simulink model "SIM_SAD_DEMO"  (R2025b)
settings: Solver=ode5  StartTime=0.0  StopTime=2*T  FixedStep=0.1  RelTol=1e-3
model workspace (MAT data in the model file):
  Pnull : Simulink.Parameter (value not decoded)
  rho_albedo_medio : Simulink.Parameter (value not decoded)
values from neighbouring files (symbols this model uses):
  Aree = zeros(10,1)    [SCRIPT_SAD_DEMO.m]
  base_seed = base_seed_MC + k    [SCRIPT_SAD_DEMO.m]
  c = astroConstants(5)*1e3    [SCRIPT_SAD_DEMO.m]
  draan = 1.99096871e-7    (= 1.99096871e-07)    [SCRIPT_SAD_DEMO.m]
  dwell_time = 30    [SCRIPT_SAD_DEMO.m]
  eps_att = deg2rad(0.2)    [SCRIPT_SAD_DEMO.m]
  eps_E = deg2rad(astroConstants(63))    [SCRIPT_SAD_DEMO.m]
  eps_h_r = 0.001    [SCRIPT_SAD_DEMO.m]
  eps_w = deg2rad(0.1)    [SCRIPT_SAD_DEMO.m]
  err_max = deg2rad(15)    [SCRIPT_SAD_DEMO.m]
  F_e = 1358    [SCRIPT_SAD_DEMO.m]
  h_r_max = 0.05    [SCRIPT_SAD_DEMO.m]
  h_r_safe = 0.001    [SCRIPT_SAD_DEMO.m]
  j_B = [0.01; 0.05; 0.01]    [SCRIPT_SAD_DEMO.m]
  J_depl = J_nom    [SCRIPT_SAD_DEMO.m]
  JD0 = juliandate(startTime)    [SCRIPT_SAD_DEMO.m]
  k_b = 200000    [SCRIPT_SAD_DEMO.m]
  Kd = K(:, 1:3)    [SCRIPT_SAD_DEMO.m]
  kep = [a,e,incl,raan,w,theta]    [SCRIPT_SAD_DEMO.m]
  Kp = K(:, 4:6)    [SCRIPT_SAD_DEMO.m]
  mu = astroConstants(13)    [SCRIPT_SAD_DEMO.m]
  n = sqrt( (mu/ (a)^3))    [SCRIPT_SAD_DEMO.m]
  n_sun = 2*pi/T_sun    (= 1.99238499086e-07)    [SCRIPT_SAD_DEMO.m]
  Nmat = [ ... (first row only)    [SCRIPT_SAD_DEMO.m]
  r_sun = 1*AU    [SCRIPT_SAD_DEMO.m]
  Re = astroConstants(23)    [SCRIPT_SAD_DEMO.m]
  rf = [ ... (first row only)    [SCRIPT_SAD_DEMO.m]
  rhod = 0.1*ones(10,1)    [SCRIPT_SAD_DEMO.m]
  rhos = zeros(10,1)    [SCRIPT_SAD_DEMO.m]
  SRP = SRP_nom    [SCRIPT_SAD_DEMO.m]
  theta = 0    [SCRIPT_SAD_DEMO.m]
  w0 = w0_nom    [SCRIPT_SAD_DEMO.m]
  w_enter = Control.w_tumbling    [SCRIPT_SAD_DEMO.m]
  w_enter_2 = Control.w_pointing    [SCRIPT_SAD_DEMO.m]
  w_exit = deg2rad(4)    [SCRIPT_SAD_DEMO.m]
  w_exit_2 = deg2rad(1.5)    [SCRIPT_SAD_DEMO.m]
symbols that are objects in the model workspace (value not decoded): Pnull, rho_albedo_medio
undefined symbols (not defined in the file or in its folder): DiscIntNeverNeededParam, Filter, Gyro, Magmeter, MTQ, q, RW, Sun_sensor
libraries: matrix_library x41, LIBRARY_SAD x40, simulink x1, cstblocks x1
(part 3 of 4)

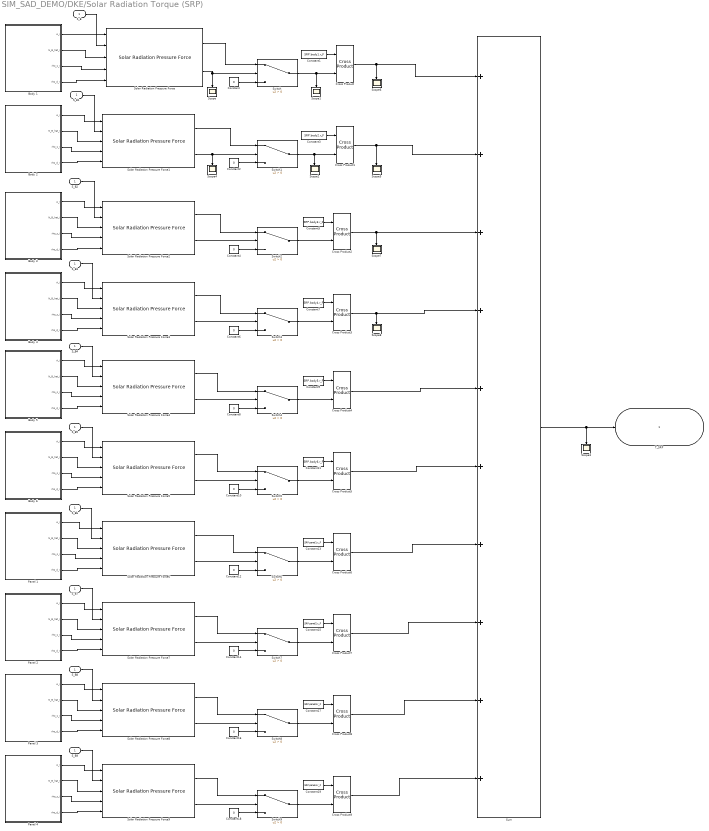
== system SIM_SAD_DEMO/DKE/Solar Radiation Torque (SRP) ==
  S_B : Inport
  Body 1 : Subsystem
  Body 2 : Subsystem
  Body 3 : Subsystem
  Body 4 : Subsystem
  Body 5 : Subsystem
  Body 6 : Subsystem
  Constant{,2,4,6,8,10,12,14,16,18} (10 alike) : Constant  Value=0
  Constant1 : Constant  Value=SRP.body1.r_F
  Constant11 : Constant  Value=SRP.body6.r_F
  Constant13 : Constant  Value=SRP.panel1.r_F
  Constant15 : Constant  Value=SRP.panel2.r_F
  Constant17 : Constant  Value=SRP.panel3.r_F
  Constant19 : Constant  Value=SRP.panel4.r_F
  Constant3 : Constant  Value=SRP.body2.r_F
  Constant5 : Constant  Value=SRP.body3.r_F
  Constant7 : Constant  Value=SRP.body4.r_F
  Constant9 : Constant  Value=SRP.body5.r_F
  Cross Product{,1..9} (10 alike) : matrix_library/Cross Product
  Panel 1 : Subsystem
  Panel 2 : Subsystem
  Panel 3 : Subsystem
  Panel 4 : Subsystem
  S_B{1..9} (9 alike) : InportShadow
  Scope{,1..8} (9 alike) : Scope
      Scope settings: ActiveDisplayYMinimum=-1  ActiveDisplayYMaximum=1  DataLoggingVariableName=ScopeData9
      Scope1 settings: ActiveDisplayYMinimum=-1  ActiveDisplayYMaximum=1  DataLoggingVariableName=ScopeData10
      Scope2 settings: ActiveDisplayYMinimum=-1  ActiveDisplayYMaximum=1  DataLoggingVariableName=ScopeData11
      Scope3 settings: ActiveDisplayYMinimum=-5.1359030627651383E-25  ActiveDisplayYMaximum=9.2718061255302776E-25  DataLoggingVariableName=ScopeData12
      Scope4 settings: ActiveDisplayYMinimum=-1  ActiveDisplayYMaximum=1  DataLoggingVariableName=ScopeData13
      Scope5 settings: ActiveDisplayYMinimum=-1  ActiveDisplayYMaximum=1  DataLoggingVariableName=ScopeData14
      Scope6 settings: ActiveDisplayYMinimum=-1  ActiveDisplayYMaximum=1  DataLoggingVariableName=ScopeData15
      Scope7 settings: ActiveDisplayYMinimum=-1  ActiveDisplayYMaximum=1  DataLoggingVariableName=ScopeData18
      Scope8 settings: ActiveDisplayYMinimum=-1  ActiveDisplayYMaximum=1  DataLoggingVariableName=ScopeData19
  Solar Radiation Pressure Force{,1..9} (10 alike) : LIBRARY_SAD/Solar Radiation Pressure Force  SystemSampleTime=-1  VariantActivationTime=update diagram  EmptyChoice=off  PassThrough=off  PassThroughVariantControl=(default)  EmptyChoiceVariantControl=(default)  AllowFlexibleInterface=on  Latency=0  AutoFrameSizeCalculation=off
  Sum : Sum  Inputs=++++++++++
  Switch{,1..9} (10 alike) : Switch  Criteria=u2 > Threshold  SaturateOnIntegerOverflow=off  InputSameDT=off
  T_SRP : Outport
  wires:
  S_B/1 -> Solar Radiation Pressure Force/2
  Body 1/1(A_i) -> Solar Radiation Pressure Force/1
  Body 1/2(N_B_hat_i) -> Solar Radiation Pressure Force/3
  Body 1/3(rho_s_i) -> Solar Radiation Pressure Force/4
  Body 1/4(rho_d_i) -> Solar Radiation Pressure Force/5
  Solar Radiation Pressure Force/1 -> Switch/1
  Solar Radiation Pressure Force/2 -> Scope/1, Switch/2
  Body 2/4(rho_d_i) -> Solar Radiation Pressure Force1/5
  Body 2/3(rho_s_i) -> Solar Radiation Pressure Force1/4
  Body 2/2(N_B_hat_i) -> Solar Radiation Pressure Force1/3
  Body 2/1(A_i) -> Solar Radiation Pressure Force1/1
  S_B1/1 -> Solar Radiation Pressure Force1/2
  S_B2/1 -> Solar Radiation Pressure Force2/2
  Body 3/1(A_i) -> Solar Radiation Pressure Force2/1
  Body 3/2(N_B_hat_i) -> Solar Radiation Pressure Force2/3
  Body 3/3(rho_s_i) -> Solar Radiation Pressure Force2/4
  Body 3/4(rho_d_i) -> Solar Radiation Pressure Force2/5
  Body 4/4(rho_d_i) -> Solar Radiation Pressure Force3/5
  Body 4/3(rho_s_i) -> Solar Radiation Pressure Force3/4
  Body 4/2(N_B_hat_i) -> Solar Radiation Pressure Force3/3
  Body 4/1(A_i) -> Solar Radiation Pressure Force3/1
  S_B3/1 -> Solar Radiation Pressure Force3/2
  S_B4/1 -> Solar Radiation Pressure Force4/2
  Body 5/1(A_i) -> Solar Radiation Pressure Force4/1
  Body 5/2(N_B_hat_i) -> Solar Radiation Pressure Force4/3
  Body 5/3(rho_s_i) -> Solar Radiation Pressure Force4/4
  Body 5/4(rho_d_i) -> Solar Radiation Pressure Force4/5
  Body 6/4(rho_d_i) -> Solar Radiation Pressure Force5/5
  Body 6/3(rho_s_i) -> Solar Radiation Pressure Force5/4
  Body 6/2(N_B_hat_i) -> Solar Radiation Pressure Force5/3
  Body 6/1(A_i) -> Solar Radiation Pressure Force5/1
  S_B5/1 -> Solar Radiation Pressure Force5/2
  S_B6/1 -> Solar Radiation Pressure Force6/2
  Panel 1/1(A_i) -> Solar Radiation Pressure Force6/1
  Panel 1/2(N_B_hat_i) -> Solar Radiation Pressure Force6/3
  Panel 1/3(rho_s_i) -> Solar Radiation Pressure Force6/4
  Panel 1/4(rho_d_i) -> Solar Radiation Pressure Force6/5
  Panel 2/4(rho_d_i) -> Solar Radiation Pressure Force7/5
  Panel 2/3(rho_s_i) -> Solar Radiation Pressure Force7/4
  Panel 2/2(N_B_hat_i) -> Solar Radiation Pressure Force7/3
  Panel 2/1(A_i) -> Solar Radiation Pressure Force7/1
  S_B7/1 -> Solar Radiation Pressure Force7/2
  S_B8/1 -> Solar Radiation Pressure Force8/2
  Panel 3/1(A_i) -> Solar Radiation Pressure Force8/1
  Panel 3/2(N_B_hat_i) -> Solar Radiation Pressure Force8/3
  Panel 3/3(rho_s_i) -> Solar Radiation Pressure Force8/4
  Panel 3/4(rho_d_i) -> Solar Radiation Pressure Force8/5
  Panel 4/4(rho_d_i) -> Solar Radiation Pressure Force9/5
  Panel 4/3(rho_s_i) -> Solar Radiation Pressure Force9/4
  Panel 4/2(N_B_hat_i) -> Solar Radiation Pressure Force9/3
  Panel 4/1(A_i) -> Solar Radiation Pressure Force9/1
  S_B9/1 -> Solar Radiation Pressure Force9/2
  Constant/1 -> Switch/3
  Switch/1 -> Scope1/1, Cross Product/2
  Constant1/1 -> Cross Product/1
  Cross Product/1 -> Scope6/1, Sum/1
  Cross Product1/1 -> Sum/2, Scope5/1
  Constant3/1 -> Cross Product1/1
  Switch1/1 -> Scope2/1, Cross Product1/2
  Constant2/1 -> Switch1/3
  Solar Radiation Pressure Force1/2 -> Scope4/1, Switch1/2
  Solar Radiation Pressure Force1/1 -> Switch1/1
  Solar Radiation Pressure Force2/1 -> Switch2/1
  Solar Radiation Pressure Force2/2 -> Switch2/2
  Constant4/1 -> Switch2/3
  Switch2/1 -> Cross Product2/2
  Constant5/1 -> Cross Product2/1
  Cross Product2/1 -> Scope7/1, Sum/3
  Cross Product3/1 -> Scope8/1, Sum/4
  Constant7/1 -> Cross Product3/1
  Switch3/1 -> Cross Product3/2
  Constant6/1 -> Switch3/3
  Solar Radiation Pressure Force3/2 -> Switch3/2
  Solar Radiation Pressure Force3/1 -> Switch3/1
  Solar Radiation Pressure Force4/1 -> Switch4/1
  Solar Radiation Pressure Force4/2 -> Switch4/2
  Constant8/1 -> Switch4/3
  Switch4/1 -> Cross Product4/2
  Constant9/1 -> Cross Product4/1
  Cross Product4/1 -> Sum/5
  Cross Product5/1 -> Sum/6
  Constant11/1 -> Cross Product5/1
  Switch5/1 -> Cross Product5/2
  Constant10/1 -> Switch5/3
  Solar Radiation Pressure Force5/2 -> Switch5/2
  Solar Radiation Pressure Force5/1 -> Switch5/1
  Solar Radiation Pressure Force6/1 -> Switch6/1
  Solar Radiation Pressure Force6/2 -> Switch6/2
  Constant12/1 -> Switch6/3
  Switch6/1 -> Cross Product6/2
  Constant13/1 -> Cross Product6/1
  Cross Product6/1 -> Sum/7
  Cross Product7/1 -> Sum/8
  Constant15/1 -> Cross Product7/1
  Switch7/1 -> Cross Product7/2
  Constant14/1 -> Switch7/3
  Solar Radiation Pressure Force7/2 -> Switch7/2
  Solar Radiation Pressure Force7/1 -> Switch7/1
  Solar Radiation Pressure Force8/1 -> Switch8/1
  Solar Radiation Pressure Force8/2 -> Switch8/2
  Constant16/1 -> Switch8/3
  Switch8/1 -> Cross Product8/2
  Constant17/1 -> Cross Product8/1
  Cross Product8/1 -> Sum/9
  Cross Product9/1 -> Sum/10
  Constant19/1 -> Cross Product9/1
  Switch9/1 -> Cross Product9/2
  Constant18/1 -> Switch9/3
  Solar Radiation Pressure Force9/2 -> Switch9/2
  Solar Radiation Pressure Force9/1 -> Switch9/1
  Sum/1 -> Scope3/1, T_SRP/1

== system SIM_SAD_DEMO/DKE/Sun-Earth Orbit ==
  Clock : Clock
  Clock1 : Clock
  Clock2 : Clock
  Constant : Constant  Value=n_sun
  Constant1 : Constant  Value=eps_E
  Constant2 : Constant  Value=r_sun
  Constant3 : Constant  Value=n_sun
  Constant4 : Constant  Value=eps_E
  Constant5 : Constant  Value=n_sun
  Cos : Trigonometry  Operator=cos
  Cos1 : Trigonometry  Operator=cos
  Cos2 : Trigonometry
  Product{,1..5} (6 alike) : Product
  Sin : Trigonometry
  Sin1 : Trigonometry
  Vector Concatenate : Concatenate  NumInputs=3
  r_Sun_N : Outport
  wires:
  Constant2/1 -> Product/1
  Clock/1 -> Product1/1
  Constant/1 -> Product1/2
  Product1/1 -> Cos/1
  Cos/1 -> Vector Concatenate/1
  Product2/1 -> Sin/1
  Constant3/1 -> Product2/2
  Clock1/1 -> Product2/1
  Sin/1 -> Product3/1
  Constant1/1 -> Cos1/1
  Product3/1 -> Vector Concatenate/2
  Cos1/1 -> Product3/2
  Cos2/1 -> Product5/2
  Product5/1 -> Vector Concatenate/3
  Constant4/1 -> Cos2/1
  Sin1/1 -> Product5/1
  Clock2/1 -> Product4/1
  Constant5/1 -> Product4/2
  Product4/1 -> Sin1/1
  Vector Concatenate/1 -> Product/2
  Product/1 -> r_Sun_N/1

== system SIM_SAD_DEMO/DKE/w_LVLH//N ==
  theta_dot : Inport
  Constant2 : Constant  Value=0
  Constant3 : Constant  Value=0
  Vector Concatenate1 : Concatenate  NumInputs=3
  Out1 : Outport
  wires:
  Vector Concatenate1/1 -> Out1/1  "w_LVLH/N"
  Constant2/1 -> Vector Concatenate1/1
  Constant3/1 -> Vector Concatenate1/2
  theta_dot/1 -> Vector Concatenate1/3

== system SIM_SAD_DEMO/SENSORS/Gyroscope ==
  note: Misalignment e non-orthogonality
  note: Scale Factor Errors
  w_B (rad/s) : Inport
  Abs : Abs  SaturateOnIntegerOverflow=off
  Bias Instability (Brown noise) : RandomNumber  Seed=base_seed + 10  SampleTime=0.2
  Constant : Constant  Value=Gyro.R
  Constant1 : Constant  Value=Gyro.O
  Constant2 : Constant  Value=Gyro.b
  Constant3 : Constant  Value=0
  D2R : Gain  Gain=pi/180
  Discrete-Time Integrator : DiscreteIntegrator  SampleTime=-1  ICPrevOutput=DiscIntNeverNeededParam  ICPrevScaledInput=DiscIntNeverNeededParam
  Gain2 : Gain  Gain=Gyro.D/(sqrt(2*Gyro.Ts))
  Gain4 : Gain  Gain=Gyro.D/(sqrt(2*Gyro.Ts))
  Gain5 : Gain  Gain=1/Gyro.ctime
  Gain6 : Gain  Gain=Gyro.NL/100
  MatrixMultiply : Product  Multiplication=Matrix(*)
  MatrixMultiply2 : Product  Multiplication=Matrix(*)
  Minus : Sum  Inputs=+-
  Plus : Sum
  Plus1 : Sum  Inputs=+++
  Plus2 : Sum
  Quantizer : Quantizer  QuantizationInterval=Gyro.LSB
  R2D : Gain  Gain=180/pi
  R2D_1 : Gain  Gain=180/pi
  Saturation : Saturate  UpperLimit=Gyro.FS/2  LowerLimit=-Gyro.FS/2
  Scope{,1..6} (7 alike) : Scope
      Scope settings: ActiveDisplayYMinimum=-1  ActiveDisplayYMaximum=1  DataLoggingVariableName=ScopeData38
      Scope1 settings: ActiveDisplayYMinimum=-1  ActiveDisplayYMaximum=1  DataLoggingVariableName=ScopeData39
      Scope2 settings: ActiveDisplayYMinimum=-1  ActiveDisplayYMaximum=1  DataLoggingVariableName=ScopeData40
      Scope3 settings: ActiveDisplayYMinimum=-1  ActiveDisplayYMaximum=1  DataLoggingVariableName=ScopeData41
      Scope4 settings: ActiveDisplayYMinimum=-1  ActiveDisplayYMaximum=1  DataLoggingVariableName=ScopeData42
      Scope5 settings: ActiveDisplayYMinimum=-0.14265311547660356  ActiveDisplayYMaximum=1.1268108470363587  DataLoggingVariableName=ScopeData43
      Scope6 settings: ActiveDisplayYMinimum=-0.12498036504591503  ActiveDisplayYMaximum=1.124997818338435  DataLoggingVariableName=ScopeData44
  Square : Math  Operator=square
  Switch : Switch  Criteria=u2 > Threshold  Threshold=2*Gyro.NL*Gyro.FS  SaturateOnIntegerOverflow=off  InputSameDT=off
  White noise : RandomNumber  Seed=base_seed + 9  SampleTime=0.2
  Zero-Order Hold : ZeroOrderHold  SampleTime=Gyro.Ts
  w_m : Outport
  wires:
  w_B (rad/s)/1 -> MatrixMultiply/2, R2D_1/1
  MatrixMultiply/1 -> MatrixMultiply2/2
  Constant/1 -> MatrixMultiply/1, Scope5/1
  Constant1/1 -> Scope6/1, MatrixMultiply2/1
  MatrixMultiply2/1 -> R2D/1
  Constant2/1 -> Plus1/1
  Plus1/1 -> Scope4/1, Quantizer/1
  Quantizer/1 -> Saturation/1
  Saturation/1 -> D2R/1
  Zero-Order Hold/1 -> w_m/1
  D2R/1 -> Zero-Order Hold/1
  White noise/1 -> Gain2/1
  Bias Instability (Brown noise)/1 -> Gain4/1
  Gain2/1 -> Plus2/1, Scope2/1
  Gain4/1 -> Minus/1
  Minus/1 -> Discrete-Time Integrator/1
  Abs/1 -> Switch/2
  Square/1 -> Gain6/1
  Gain6/1 -> Switch/1
  Constant3/1 -> Switch/3
  R2D_1/1 -> Abs/1, Square/1
  Switch/1 -> Scope1/1, Plus/2
  Gain5/1 -> Minus/2
  Plus2/1 -> Scope3/1, Plus1/3
  Discrete-Time Integrator/1 -> Plus2/2, Gain5/1
  Plus/1 -> Plus1/2
  R2D/1 -> Plus/1, Scope/1

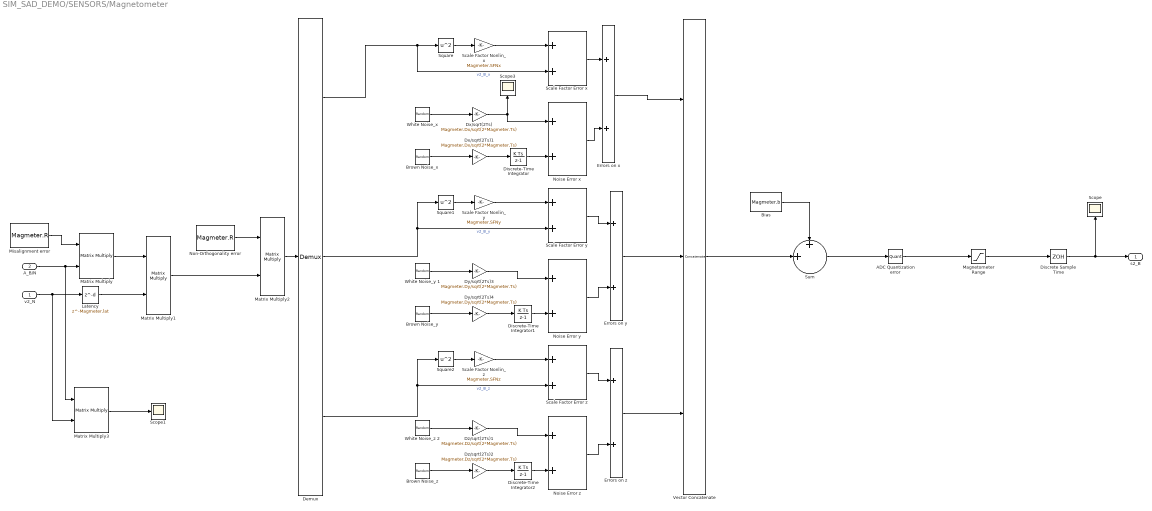
== system SIM_SAD_DEMO/SENSORS/Magnetometer ==
  v2_N : Inport
  A_B/N : Inport  Port=2
  ADC Quantization error : Quantizer  QuantizationInterval=Magmeter.LSB
  Bias : Constant  Value=Magmeter.b
  Brown Noise_x : RandomNumber  Seed=base_seed + 4  SampleTime=0.1
  Brown Noise_y : RandomNumber  Seed=base_seed + 6  SampleTime=0.1
  Brown Noise_z : RandomNumber  Seed=base_seed + 8  SampleTime=0.1
  Demux : Demux  Outputs=3
  Discrete Sample Time : ZeroOrderHold  SampleTime=Magmeter.Ts
  Discrete-Time Integrator : DiscreteIntegrator  SampleTime=-1  ICPrevOutput=DiscIntNeverNeededParam  ICPrevScaledInput=DiscIntNeverNeededParam
  Discrete-Time Integrator1 : DiscreteIntegrator  SampleTime=-1  ICPrevOutput=DiscIntNeverNeededParam  ICPrevScaledInput=DiscIntNeverNeededParam
  Discrete-Time Integrator2 : DiscreteIntegrator  SampleTime=-1  ICPrevOutput=DiscIntNeverNeededParam  ICPrevScaledInput=DiscIntNeverNeededParam
  Dx/sqrt(2Ts) : Gain  Gain=Magmeter.Dx/sqrt(2*Magmeter.Ts)
  Dx/sqrt(2Ts)1 : Gain  Gain=Magmeter.Dx/sqrt(2*Magmeter.Ts)
  Dy/sqrt(2Ts)3 : Gain  Gain=Magmeter.Dy/sqrt(2*Magmeter.Ts)
  Dy/sqrt(2Ts)4 : Gain  Gain=Magmeter.Dy/sqrt(2*Magmeter.Ts)
  Dz/sqrt(2Ts)1 : Gain  Gain=Magmeter.Dz/sqrt(2*Magmeter.Ts)
  Dz/sqrt(2Ts)2 : Gain  Gain=Magmeter.Dz/sqrt(2*Magmeter.Ts)
  Errors on x : Sum
  Errors on y : Sum
  Errors on z : Sum
  Latency : Delay  DelayLength=Magmeter.lat
  Magnetometer Range : Saturate  UpperLimit=Magmeter.FS(2)  LowerLimit=Magmeter.FS(1)
  Matrix Multiply{,1..3} (4 alike) : Product  Multiplication=Matrix(*)
  Misalignment error : Constant  Value=Magmeter.R
  Noise Error x : Sum
  Noise Error y : Sum
  Noise Error z : Sum
  Non-Orthogonality error : Constant  Value=Magmeter.R
  Scale Factor Error x : Sum
  Scale Factor Error y : Sum
  Scale Factor Error z : Sum
  Scale Factor Nonlin_x : Gain  Gain=Magmeter.SFNx
  Scale Factor Nonlin_y : Gain  Gain=Magmeter.SFNy
  Scale Factor Nonlin_z : Gain  Gain=Magmeter.SFNz
  Scope : Scope
      settings: ActiveDisplayYMinimum=-2.19268798828125E-5  ActiveDisplayYMaximum=3.19366455078125E-5  DataLoggingVariableName=ScopeData41
  Scope1 : Scope
      settings: ActiveDisplayYMinimum=-2.3197965857438213E-5  ActiveDisplayYMaximum=2.9408763146413098E-5  DataLoggingVariableName=ScopeData51
  Scope3 : Scope
      settings: ActiveDisplayYMinimum=-2.2049299467588538E-7  ActiveDisplayYMaximum=2.2303254095659386E-7  DataLoggingVariableName=ScopeData59
  Square : Math  Operator=square
  Square1 : Math  Operator=square
  Square2 : Math  Operator=square
  Sum : Sum  Inputs=++|
  Vector Concatenate : Concatenate  NumInputs=3
  "White Noise_x " : RandomNumber  Seed=base_seed + 3  SampleTime=0.1
  White Noise_y 1 : RandomNumber  Seed=base_seed + 5  SampleTime=0.1
  White Noise_z 2 : RandomNumber  Seed=base_seed + 7  SampleTime=0.1
  s2_B : Outport
  wires:
  v2_N/1 -> Matrix Multiply3/2, Latency/1
  A_B/N/1 -> Matrix Multiply3/1, Matrix Multiply/2
  Matrix Multiply/1 -> Matrix Multiply1/1
  Misalignment error/1 -> Matrix Multiply/1
  Latency/1 -> Matrix Multiply1/2
  Matrix Multiply1/1 -> Matrix Multiply2/2
  Non-Orthogonality error/1 -> Matrix Multiply2/1
  Matrix Multiply2/1 -> Demux/1
  Demux/1 -> Square/1, Scale Factor Error x/2  "v2_B_x"
  Demux/2 -> Square1/1, Scale Factor Error y/2  "v2_B_y"
  "White Noise_x "/1 -> Dx/sqrt(2Ts)/1
  Square/1 -> Scale Factor Nonlin_x/1
  Scale Factor Nonlin_x/1 -> Scale Factor Error x/1
  Noise Error x/1 -> Errors on x/2
  Scale Factor Error x/1 -> Errors on x/1
  Bias/1 -> Sum/1
  Errors on x/1 -> Vector Concatenate/1
  Vector Concatenate/1 -> Sum/2
  Sum/1 -> ADC Quantization error/1
  ADC Quantization error/1 -> Magnetometer Range/1
  Magnetometer Range/1 -> Discrete Sample Time/1
  Discrete Sample Time/1 -> s2_B/1, Scope/1
  Brown Noise_x/1 -> Dx/sqrt(2Ts)1/1
  Discrete-Time Integrator/1 -> Noise Error x/2
  Dx/sqrt(2Ts)1/1 -> Discrete-Time Integrator/1
  Demux/3 -> Scale Factor Error z/2, Square2/1  "v2_B_z"
  Dy/sqrt(2Ts)4/1 -> Discrete-Time Integrator1/1
  Discrete-Time Integrator1/1 -> Noise Error y/2
  Brown Noise_y/1 -> Dy/sqrt(2Ts)4/1
  Errors on y/1 -> Vector Concatenate/2
  Dy/sqrt(2Ts)3/1 -> Noise Error y/1
  Scale Factor Error y/1 -> Errors on y/1
  Noise Error y/1 -> Errors on y/2
  Scale Factor Nonlin_y/1 -> Scale Factor Error y/1
  Square1/1 -> Scale Factor Nonlin_y/1
  White Noise_y 1/1 -> Dy/sqrt(2Ts)3/1
  White Noise_z 2/1 -> Dz/sqrt(2Ts)1/1
  Square2/1 -> Scale Factor Nonlin_z/1
  Scale Factor Nonlin_z/1 -> Scale Factor Error z/1
  Noise Error z/1 -> Errors on z/2
  Scale Factor Error z/1 -> Errors on z/1
  Dz/sqrt(2Ts)1/1 -> Noise Error z/1
  Errors on z/1 -> Vector Concatenate/3
  Brown Noise_z/1 -> Dz/sqrt(2Ts)2/1
  Discrete-Time Integrator2/1 -> Noise Error z/2
  Dz/sqrt(2Ts)2/1 -> Discrete-Time Integrator2/1
  Matrix Multiply3/1 -> Scope1/1
  Dx/sqrt(2Ts)/1 -> Scope3/1, Noise Error x/1

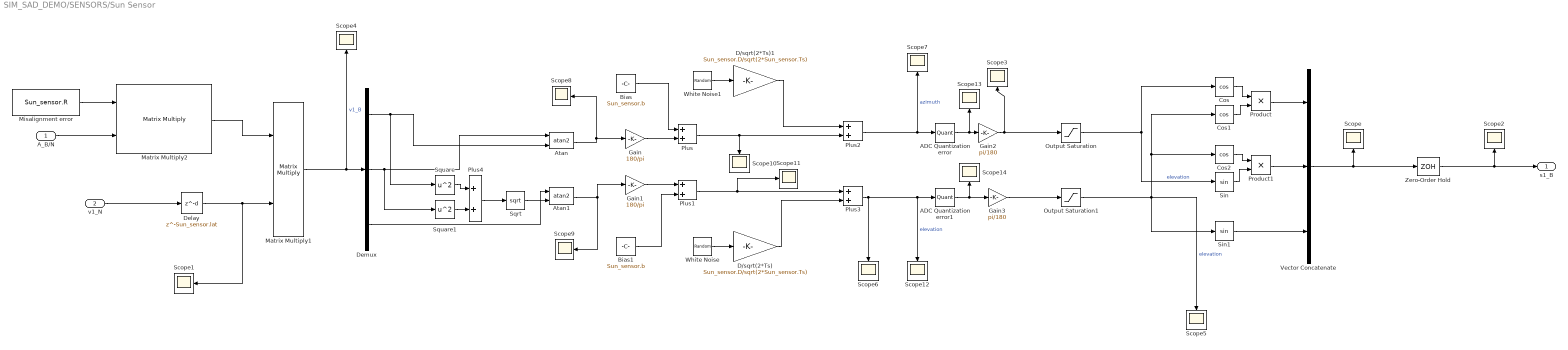
== system SIM_SAD_DEMO/SENSORS/Sun Sensor ==
  A_B/N : Inport
  v1_N : Inport  Port=2
  ADC Quantization error : Quantizer  QuantizationInterval=Sun_sensor.LSB
  ADC Quantization error1 : Quantizer  QuantizationInterval=Sun_sensor.LSB
  Atan : Trigonometry  Operator=atan2
  Atan1 : Trigonometry  Operator=atan2
  Bias : Constant  Value=Sun_sensor.b
  Bias1 : Constant  Value=Sun_sensor.b
  Cos : Trigonometry  Operator=cos
  Cos1 : Trigonometry  Operator=cos
  Cos2 : Trigonometry  Operator=cos
  D/sqrt(2*Ts) : Gain  Gain=Sun_sensor.D/sqrt(2*Sun_sensor.Ts)
  D/sqrt(2*Ts)1 : Gain  Gain=Sun_sensor.D/sqrt(2*Sun_sensor.Ts)
  Delay : Delay  DelayLength=Sun_sensor.lat
  Demux : Demux  Outputs=3
  Gain : Gain  Gain=180/pi
  Gain1 : Gain  Gain=180/pi
  Gain2 : Gain  Gain=pi/180
  Gain3 : Gain  Gain=pi/180
  Matrix Multiply1 : Product  Multiplication=Matrix(*)
  Matrix Multiply2 : Product  Multiplication=Matrix(*)
  Misalignment error : Constant  Value=Sun_sensor.R
  Output Saturation : Saturate  UpperLimit=Sun_sensor.FOV(2)  LowerLimit=Sun_sensor.FOV(1)
  Output Saturation1 : Saturate  UpperLimit=Sun_sensor.FOV(2)  LowerLimit=Sun_sensor.FOV(1)
  Plus{,1..4} (5 alike) : Sum
  Product : Product
  Product1 : Product
  Scope{,1..14} (15 alike) : Scope
      Scope settings: ActiveDisplayYMinimum=-1.2499999209761798  ActiveDisplayYMaximum=1.2499998658254696  DataLoggingVariableName=ScopeData38
      Scope1 settings: ActiveDisplayYMinimum=-0.50368682988878122  ActiveDisplayYMaximum=0.83961433978529221  DataLoggingVariableName=ScopeData39
      Scope10 settings: ActiveDisplayYMinimum=-1  ActiveDisplayYMaximum=1  DataLoggingVariableName=ScopeData48
      Scope11 settings: ActiveDisplayYMinimum=-0.16263647893928282  ActiveDisplayYMaximum=0.22803548611194213  DataLoggingVariableName=ScopeData49
      Scope12 settings: ActiveDisplayYMinimum=-1  ActiveDisplayYMaximum=1  DataLoggingVariableName=ScopeData50
      Scope13 settings: ActiveDisplayYMinimum=-225.30372619628906  ActiveDisplayYMaximum=225.44471740722656  DataLoggingVariableName=ScopeData53
      Scope14 settings: ActiveDisplayYMinimum=-0.908203125  ActiveDisplayYMaximum=0.95947265625  DataLoggingVariableName=ScopeData54
      Scope2 settings: ActiveDisplayYMinimum=-1.0615675808468883  ActiveDisplayYMaximum=1.1316838676859093  DataLoggingVariableName=ScopeData40
      Scope3 settings: ActiveDisplayYMinimum=-3.91845703125  ActiveDisplayYMaximum=3.91845703125  DataLoggingVariableName=ScopeData43
      Scope4 settings: ActiveDisplayYMinimum=-1.2500019852403355  ActiveDisplayYMaximum=1.2500020169480639  DataLoggingVariableName=ScopeData42
      Scope5 settings: ActiveDisplayYMinimum=-0.015851134808151625  ActiveDisplayYMaximum=0.01674595693441825  DataLoggingVariableName=ScopeData52
      Scope6 settings: ActiveDisplayYMinimum=-1  ActiveDisplayYMaximum=1  DataLoggingVariableName=ScopeData44
      Scope7 settings: ActiveDisplayYMinimum=-225.01352290442006  ActiveDisplayYMaximum=225.27088940788934  DataLoggingVariableName=ScopeData45
      Scope8 settings: ActiveDisplayYMinimum=-3.6715953390719882  ActiveDisplayYMaximum=3.318983817677017  DataLoggingVariableName=ScopeData46
      Scope9 settings: ActiveDisplayYMinimum=-1  ActiveDisplayYMaximum=1  DataLoggingVariableName=ScopeData47
  Sin : Trigonometry
  Sin1 : Trigonometry
  Sqrt : Sqrt
  Square : Math  Operator=square
  Square1 : Math  Operator=square
  Vector Concatenate : Concatenate  NumInputs=3
  White Noise : RandomNumber  Seed=base_seed + 2  SampleTime=0.1
  White Noise1 : RandomNumber  Seed=base_seed + 1  SampleTime=0.1
  Zero-Order Hold : ZeroOrderHold  SampleTime=Sun_sensor.Ts
  s1_B : Outport
  wires:
  A_B/N/1 -> Matrix Multiply2/2
  Zero-Order Hold/1 -> s1_B/1, Scope2/1
  Vector Concatenate/1 -> Zero-Order Hold/1, Scope/1
  v1_N/1 -> Delay/1
  Misalignment error/1 -> Matrix Multiply2/1
  White Noise/1 -> D/sqrt(2*Ts)/1
  Bias/1 -> Plus/1
  Matrix Multiply1/1 -> Scope4/1, Demux/1  "v1_B"
  Atan/1 -> Scope8/1, Gain/1
  Atan1/1 -> Gain1/1, Scope9/1
  Delay/1 -> Matrix Multiply1/2, Scope1/1
  Gain/1 -> Plus/2
  Gain1/1 -> Plus1/1
  Plus/1 -> Plus2/2, Scope10/1
  Plus1/1 -> Scope11/1, Plus3/1
  D/sqrt(2*Ts)/1 -> Plus3/2
  Bias1/1 -> Plus1/2
  White Noise1/1 -> D/sqrt(2*Ts)1/1
  D/sqrt(2*Ts)1/1 -> Plus2/1
  Demux/3 -> Atan1/1
  Demux/1 -> Square/1, Atan/2
  Product/1 -> Vector Concatenate/1
  Demux/2 -> Square1/1, Atan/1
  Square1/1 -> Plus4/2
  Square/1 -> Plus4/1
  Plus4/1 -> Sqrt/1
  Sqrt/1 -> Atan1/2
  Cos/1 -> Product/1
  Cos1/1 -> Product/2
  ADC Quantization error/1 -> Gain2/1, Scope13/1
  ADC Quantization error1/1 -> Gain3/1, Scope14/1
  Sin1/1 -> Vector Concatenate/3
  Cos2/1 -> Product1/1
  Sin/1 -> Product1/2
  Product1/1 -> Vector Concatenate/2
  Plus3/1 -> Scope6/1, ADC Quantization error1/1, Scope12/1  "elevation"
  Plus2/1 -> ADC Quantization error/1, Scope7/1  "azimuth"
  Matrix Multiply2/1 -> Matrix Multiply1/1
  Gain2/1 -> Scope3/1, Output Saturation/1
  Gain3/1 -> Output Saturation1/1
  Output Saturation/1 -> Cos/1, Sin/1  "elevation"
  Output Saturation1/1 -> Scope5/1, Cos2/1, Cos1/1, Sin1/1  "elevation"

== system SIM_SAD_DEMO/q-->DCM/[qΛ] ==
  q : Inport
  Constant : Constant  Value=0
  Constant1 : Constant  Value=0
  Constant2 : Constant  Value=0
  Demux : Demux
  Gain : Gain  Gain=-1
  Gain1 : Gain  Gain=-1
  Gain2 : Gain  Gain=-1
  Terminator : Terminator
  Vector Concatenate : Concatenate  NumInputs=3
  Vector Concatenate1 : Concatenate  NumInputs=3  Mode=Multidimensional array  ConcatenateDimension=2
  Vector Concatenate2 : Concatenate  NumInputs=3
  Vector Concatenate3 : Concatenate  NumInputs=3
  "[qΛ]" : Outport
  wires:
  q/1 -> Demux/1
  Demux/1 -> Gain2/1, Vector Concatenate2/3  "q1"
  Demux/2 -> Vector Concatenate3/1, Gain/1  "q2"
  Demux/3 -> Vector Concatenate/2, Gain1/1  "q3"
  Demux/4 -> Terminator/1  "q4"
  Constant/1 -> Vector Concatenate/1
  Gain/1 -> Vector Concatenate/3
  Vector Concatenate/1 -> Vector Concatenate1/1
  Constant1/1 -> Vector Concatenate2/2
  Gain1/1 -> Vector Concatenate2/1
  Vector Concatenate2/1 -> Vector Concatenate1/2
  Gain2/1 -> Vector Concatenate3/2
  Constant2/1 -> Vector Concatenate3/3
  Vector Concatenate3/1 -> Vector Concatenate1/3
  Vector Concatenate1/1 -> "[qΛ]"/1

== system SIM_SAD_DEMO/q-->DCM1/[qΛ] ==
  q : Inport
  Constant : Constant  Value=0
  Constant1 : Constant  Value=0
  Constant2 : Constant  Value=0
  Demux : Demux
  Gain : Gain  Gain=-1
  Gain1 : Gain  Gain=-1
  Gain2 : Gain  Gain=-1
  Terminator : Terminator
  Vector Concatenate : Concatenate  NumInputs=3
  Vector Concatenate1 : Concatenate  NumInputs=3  Mode=Multidimensional array  ConcatenateDimension=2
  Vector Concatenate2 : Concatenate  NumInputs=3
  Vector Concatenate3 : Concatenate  NumInputs=3
  "[qΛ]" : Outport
  wires:
  q/1 -> Demux/1
  Demux/1 -> Gain2/1, Vector Concatenate2/3  "q1"
  Demux/2 -> Vector Concatenate3/1, Gain/1  "q2"
  Demux/3 -> Vector Concatenate/2, Gain1/1  "q3"
  Demux/4 -> Terminator/1  "q4"
  Constant/1 -> Vector Concatenate/1
  Gain/1 -> Vector Concatenate/3
  Vector Concatenate/1 -> Vector Concatenate1/1
  Constant1/1 -> Vector Concatenate2/2
  Gain1/1 -> Vector Concatenate2/1
  Vector Concatenate2/1 -> Vector Concatenate1/2
  Gain2/1 -> Vector Concatenate3/2
  Constant2/1 -> Vector Concatenate3/3
  Vector Concatenate3/1 -> Vector Concatenate1/3
  Vector Concatenate1/1 -> "[qΛ]"/1

== system SIM_SAD_DEMO/ACTUATORS/Detumbling (MTQ only)/Norm1 ==
  note: square
  In1 : Inport
  Sqrt : Sqrt
  Square1 : Math  Operator=square
  Sum of Elements : Sum  Inputs=+
  Out1 : Outport
  wires:
  Sum of Elements/1 -> Sqrt/1
  In1/1 -> Square1/1
  Sqrt/1 -> Out1/1
  Square1/1 -> Sum of Elements/1

== system SIM_SAD_DEMO/ACTUATORS/Slew//tracking (MTQ + RW)/A* (pseudo-inverse) ==
  Constant : Constant  Value=RW.A
  Constant1 : Constant  Value=RW.A
  Constant2 : Constant  Value=RW.A
  Matrix Divide : Product  Inputs=/  Multiplication=Matrix(*)
  MatrixMultiply : Product  Multiplication=Matrix(*)
  MatrixMultiply1 : Product  Multiplication=Matrix(*)
  Transpose : Math  Operator=transpose
  Transpose1 : Math  Operator=transpose
  A* : Outport
  wires:
  Constant/1 -> Transpose/1
  Transpose/1 -> MatrixMultiply/1
  Constant1/1 -> MatrixMultiply/2
  MatrixMultiply/1 -> Matrix Divide/1
  Matrix Divide/1 -> MatrixMultiply1/1
  Constant2/1 -> Transpose1/1
  Transpose1/1 -> MatrixMultiply1/2
  MatrixMultiply1/1 -> A*/1

== system SIM_SAD_DEMO/ACTUATORS/Slew//tracking (MTQ + RW)/Norm1 ==
  note: square
  In1 : Inport
  Sqrt : Sqrt
  Square1 : Math  Operator=square
  Sum of Elements : Sum  Inputs=+
  Out1 : Outport
  wires:
  Sum of Elements/1 -> Sqrt/1
  In1/1 -> Square1/1
  Sqrt/1 -> Out1/1
  Square1/1 -> Sum of Elements/1

== system SIM_SAD_DEMO/ATTITUDE DETERMINATION (q-method)/w_est (q)/Normalized Vector ==
  r : Inport
  Divide : Product  Inputs=*/
  vector_norm : LIBRARY_SAD/vector_norm  SystemSampleTime=-1  VariantActivationTime=update diagram  EmptyChoice=off  PassThrough=off  PassThroughVariantControl=(default)  EmptyChoiceVariantControl=(default)  AllowFlexibleInterface=on  Latency=0  AutoFrameSizeCalculation=off
  s1_B : Outport
  wires:
  Divide/1 -> s1_B/1
  r/1 -> Divide/1, vector_norm/1
  vector_norm/1 -> Divide/2

== system SIM_SAD_DEMO/DCM ---> q/q-->DCM (CHECK)/[qΛ] ==
  q : Inport
  Constant : Constant  Value=0
  Constant1 : Constant  Value=0
  Constant2 : Constant  Value=0
  Demux : Demux
  Gain : Gain  Gain=-1
  Gain1 : Gain  Gain=-1
  Gain2 : Gain  Gain=-1
  Terminator : Terminator
  Vector Concatenate : Concatenate  NumInputs=3
  Vector Concatenate1 : Concatenate  NumInputs=3  Mode=Multidimensional array  ConcatenateDimension=2
  Vector Concatenate2 : Concatenate  NumInputs=3
  Vector Concatenate3 : Concatenate  NumInputs=3
  "[qΛ]" : Outport
  wires:
  Vector Concatenate1/1 -> "[qΛ]"/1
  Vector Concatenate3/1 -> Vector Concatenate1/3
  Constant2/1 -> Vector Concatenate3/3
  Gain2/1 -> Vector Concatenate3/2
  Vector Concatenate2/1 -> Vector Concatenate1/2
  Gain1/1 -> Vector Concatenate2/1
  Constant1/1 -> Vector Concatenate2/2
  Vector Concatenate/1 -> Vector Concatenate1/1
  Gain/1 -> Vector Concatenate/3
  Constant/1 -> Vector Concatenate/1
  Demux/4 -> Terminator/1  "q4"
  Demux/3 -> Gain1/1, Vector Concatenate/2  "q3"
  Demux/2 -> Gain/1, Vector Concatenate3/1  "q2"
  Demux/1 -> Vector Concatenate2/3, Gain2/1  "q1"
  q/1 -> Demux/1

== system SIM_SAD_DEMO/DKE/ALBEDO_TORQUE/For Each Subsystem1 ==
  note: nelle proprietà lascio direttamente così almeno posso processare una alla volta le singole righe e colonne sia in dimension che in width
  In1 : Inport  Partition=on  PartitionDimension=1  PartitionWidth=1  PartitionOffset=0
  In2 : Inport  Port=2  Partition=on  PartitionDimension=1  PartitionWidth=1  PartitionOffset=0
  Cross Product : matrix_library/Cross Product
  For Each : ForEach  DisableCoverage=on
  Signal Specification : SignalSpecification  Dimensions=[1 3]
  Transpose : Math  Operator=transpose
  Transpose1 : Math  Operator=transpose
  Transpose2 : Math  Operator=transpose
  Out1 : Outport  ConcatenationDimension=1
  wires:
  In2/1 -> Transpose/1  "Rfi"
  In1/1 -> Transpose1/1  "Fi"
  Transpose/1 -> Cross Product/1
  Transpose1/1 -> Cross Product/2
  Cross Product/1 -> Transpose2/1
  Transpose2/1 -> Signal Specification/1
  Signal Specification/1 -> Out1/1

== system SIM_SAD_DEMO/DKE/ALBEDO_TORQUE/Normalization ==
  In1 : Inport
  Divide : Product  Inputs=*/
  Dot Product : DotProduct  OutDataTypeStr=Inherit: Inherit via internal rule
  Sqrt : Sqrt
  Out1 : Outport
  wires:
  Dot Product/1 -> Sqrt/1
  In1/1 -> Divide/1, Dot Product/2, Dot Product/1
  Divide/1 -> Out1/1
  Sqrt/1 -> Divide/2

== system SIM_SAD_DEMO/DKE/ALBEDO_TORQUE/Normalization  ==
  In1 : Inport
  Divide : Product  Inputs=*/
  Dot Product : DotProduct  OutDataTypeStr=Inherit: Inherit via internal rule
  Sqrt : Sqrt
  Out1 : Outport
  wires:
  Dot Product/1 -> Sqrt/1
  In1/1 -> Divide/1, Dot Product/2, Dot Product/1
  Divide/1 -> Out1/1
  Sqrt/1 -> Divide/2

== system SIM_SAD_DEMO/DKE/ALBEDO_TORQUE/Normalization1 ==
  R_N : Inport
  Divide : Product  Inputs=*/
  Dot Product : DotProduct  OutDataTypeStr=Inherit: Inherit via internal rule
  Sqrt : Sqrt
  Out1 : Outport
  wires:
  Dot Product/1 -> Sqrt/1
  R_N/1 -> Divide/1, Dot Product/2, Dot Product/1
  Divide/1 -> Out1/1
  Sqrt/1 -> Divide/2

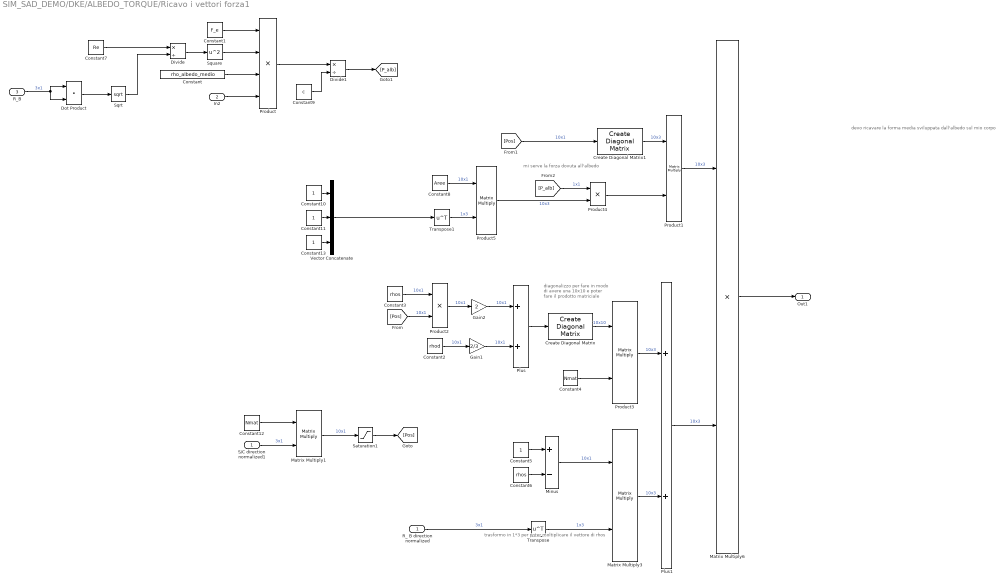
== system SIM_SAD_DEMO/DKE/ALBEDO_TORQUE/Ricavo i vettori forza1 ==
  note: devo ricavare la forma media sviluppata dall'albedo sul mio corpo
  note: mi serve la forza dovuta all'albedo
  note: diagonalizzo per fare in modo di avere una 10x10 e poter fare il prodotto matriciale
  note: trasformo in 1*3 per poter moltiplicare il vettore di rhos
  " R_ B direction normalized" : Inport
  In2 : Inport  Port=2
  R_B : Inport  Port=3
  Constant : Constant  Value=rho_albedo_medio
  Constant1 : Constant  Value=F_e
  Constant{5,10..11,13} (4 alike) : Constant
  Constant12 : Constant  Value=Nmat
  Constant2 : Constant  Value=rhod
  Constant3 : Constant  Value=rhos
  Constant4 : Constant  Value=Nmat
  Constant6 : Constant  Value=rhos
  Constant7 : Constant  Value=Re
  Constant8 : Constant  Value=Aree
  Constant9 : Constant  Value=c
  Create Diagonal Matrix : matrix_library/Create Diagonal Matrix
      settings: LibrarySourceBlock=|
      | simulink/Matrix
      | Operations/Create Diagonal
      | Matrix
  Create Diagonal Matrix1 : matrix_library/Create Diagonal Matrix
      settings: LibrarySourceBlock=|
      | simulink/Matrix
      | Operations/Create Diagonal
      | Matrix
  Divide : Product  Inputs=*/
  Divide1 : Product  Inputs=*/
  Dot Product : DotProduct  OutDataTypeStr=Inherit: Inherit via internal rule
  Gain1 : Gain  Gain=2/3
  Gain2 : Gain  Gain=2
  Matrix Multiply1 : Product  Multiplication=Matrix(*)
  Matrix Multiply3 : Product  Multiplication=Matrix(*)
  Matrix Multiply6 : Product
  Minus : Sum  Inputs=+-
  Plus : Sum
  Plus1 : Sum
  Product : Product  Inputs=4
  Product1 : Product  Multiplication=Matrix(*)
  Product2 : Product
  Product3 : Product  Multiplication=Matrix(*)
  Product4 : Product
  Product5 : Product  Multiplication=Matrix(*)
  S/C direction normalized1 : InportShadow
  Saturation1 : Saturate  UpperLimit=inf  LowerLimit=0
  Sqrt : Sqrt
  Square : Math  Operator=square
  Transpose : Math  Operator=transpose
  Transpose1 : Math  Operator=transpose
  Vector Concatenate : Concatenate  NumInputs=3
  Out1 : Outport
  wires:
  Gain1/1 -> Plus/2  "10x1"
  Plus1/1 -> Matrix Multiply6/2  "10x3"
  Product3/1 -> Plus1/1  "10x3"
  Constant4/1 -> Product3/2
  Product2/1 -> Gain2/1  "10x1"
  Constant2/1 -> Gain1/1  "10x1"
  Constant6/1 -> Minus/2
  Constant3/1 -> Product2/1  "10x1"
  Product1/1 -> Matrix Multiply6/1  "10x3"
  Gain2/1 -> Plus/1  "10x1"
  " R_ B direction normalized"/1 -> Transpose/1  "3x1"
  Matrix Multiply3/1 -> Plus1/2  "10x3"
  Constant5/1 -> Minus/1
  Matrix Multiply6/1 -> Out1/1
  [Pos] -> Create Diagonal Matrix1/1  "10x1"
  Matrix Multiply1/1 -> Saturation1/1  "10x1"
  Constant12/1 -> Matrix Multiply1/1
  Minus/1 -> Matrix Multiply3/1  "10x1"
  Transpose/1 -> Matrix Multiply3/2  "1x3"
  Saturation1/1 -> [Pos]
  [Pos] -> Product2/2  "10x1"
  Plus/1 -> Create Diagonal Matrix/1
  Constant13/1 -> Vector Concatenate/3
  Constant10/1 -> Vector Concatenate/1
  Constant11/1 -> Vector Concatenate/2
  Vector Concatenate/1 -> Transpose1/1
  Create Diagonal Matrix/1 -> Product3/1  "10x10"
  Transpose1/1 -> Product5/2  "1x3"
  Constant8/1 -> Product5/1  "10x1"
  Product5/1 -> Product4/2  "10x3"
  Create Diagonal Matrix1/1 -> Product1/1  "10x3"
  Product4/1 -> Product1/2
  S/C direction normalized1/1 -> Matrix Multiply1/2  "3x1"
  Constant7/1 -> Divide/1
  Divide/1 -> Square/1
  Constant1/1 -> Product/1
  Square/1 -> Product/2
  Constant/1 -> Product/3
  In2/1 -> Product/4
  Product/1 -> Divide1/1
  Constant9/1 -> Divide1/2
  Divide1/1 -> [P_alb]
  [P_alb] -> Product4/1  "1x1"
  Sqrt/1 -> Divide/2
  R_B/1 -> Dot Product/1, Dot Product/2  "3x1"
  Dot Product/1 -> Sqrt/1

== system SIM_SAD_DEMO/DKE/Earth radiation torque/Body 1 ==
  Constant : Constant  Value=SRP.body1.A
  Constant1 : Constant  Value=SRP.body1.N_hat
  Constant2 : Constant  Value=SRP.body1.rho_s
  Constant3 : Constant  Value=SRP.body1.rho_d
  A_i : Outport
  N_B_hat_i : Outport  Port=2
  rho_s_i : Outport  Port=3
  rho_d_i : Outport  Port=4
  wires:
  Constant/1 -> A_i/1
  Constant1/1 -> N_B_hat_i/1
  Constant2/1 -> rho_s_i/1
  Constant3/1 -> rho_d_i/1

== system SIM_SAD_DEMO/DKE/Earth radiation torque/Body 2 ==
  Constant : Constant  Value=SRP.body2.A
  Constant1 : Constant  Value=SRP.body2.N_hat
  Constant2 : Constant  Value=SRP.body2.rho_s
  Constant3 : Constant  Value=SRP.body2.rho_d
  A_i : Outport
  N_B_hat_i : Outport  Port=2
  rho_s_i : Outport  Port=3
  rho_d_i : Outport  Port=4
  wires:
  Constant3/1 -> rho_d_i/1
  Constant2/1 -> rho_s_i/1
  Constant1/1 -> N_B_hat_i/1
  Constant/1 -> A_i/1

== system SIM_SAD_DEMO/DKE/Earth radiation torque/Body 3 ==
  Constant : Constant  Value=SRP.body3.A
  Constant1 : Constant  Value=SRP.body3.N_hat
  Constant2 : Constant  Value=SRP.body3.rho_s
  Constant3 : Constant  Value=SRP.body3.rho_d
  A_i : Outport
  N_B_hat_i : Outport  Port=2
  rho_s_i : Outport  Port=3
  rho_d_i : Outport  Port=4
  wires:
  Constant/1 -> A_i/1
  Constant1/1 -> N_B_hat_i/1
  Constant2/1 -> rho_s_i/1
  Constant3/1 -> rho_d_i/1

== system SIM_SAD_DEMO/DKE/Earth radiation torque/Body 4 ==
  Constant : Constant  Value=SRP.body4.A
  Constant1 : Constant  Value=SRP.body4.N_hat
  Constant2 : Constant  Value=SRP.body4.rho_s
  Constant3 : Constant  Value=SRP.body4.rho_d
  A_i : Outport
  N_B_hat_i : Outport  Port=2
  rho_s_i : Outport  Port=3
  rho_d_i : Outport  Port=4
  wires:
  Constant3/1 -> rho_d_i/1
  Constant2/1 -> rho_s_i/1
  Constant1/1 -> N_B_hat_i/1
  Constant/1 -> A_i/1

== system SIM_SAD_DEMO/DKE/Earth radiation torque/Body 5 ==
  Constant : Constant  Value=SRP.body5.A
  Constant1 : Constant  Value=SRP.body5.N_hat
  Constant2 : Constant  Value=SRP.body5.rho_s
  Constant3 : Constant  Value=SRP.body5.rho_d
  A_i : Outport
  N_B_hat_i : Outport  Port=2
  rho_s_i : Outport  Port=3
  rho_d_i : Outport  Port=4
  wires:
  Constant/1 -> A_i/1
  Constant1/1 -> N_B_hat_i/1
  Constant2/1 -> rho_s_i/1
  Constant3/1 -> rho_d_i/1

== system SIM_SAD_DEMO/DKE/Earth radiation torque/Body 6 ==
  Constant : Constant  Value=SRP.body6.A
  Constant1 : Constant  Value=SRP.body6.N_hat
  Constant2 : Constant  Value=SRP.body6.rho_s
  Constant3 : Constant  Value=SRP.body6.rho_d
  A_i : Outport
  N_B_hat_i : Outport  Port=2
  rho_s_i : Outport  Port=3
  rho_d_i : Outport  Port=4
  wires:
  Constant3/1 -> rho_d_i/1
  Constant2/1 -> rho_s_i/1
  Constant1/1 -> N_B_hat_i/1
  Constant/1 -> A_i/1

== system SIM_SAD_DEMO/DKE/Earth radiation torque/Panel 1 ==
  Constant : Constant  Value=SRP.panel1.A
  Constant1 : Constant  Value=SRP.panel1.N_hat
  Constant2 : Constant  Value=SRP.panel1.rho_s
  Constant3 : Constant  Value=SRP.panel1.rho_d
  A_i : Outport
  N_B_hat_i : Outport  Port=2
  rho_s_i : Outport  Port=3
  rho_d_i : Outport  Port=4
  wires:
  Constant/1 -> A_i/1
  Constant1/1 -> N_B_hat_i/1
  Constant2/1 -> rho_s_i/1
  Constant3/1 -> rho_d_i/1

== system SIM_SAD_DEMO/DKE/Earth radiation torque/Panel 2 ==
  Constant : Constant  Value=SRP.panel2.A
  Constant1 : Constant  Value=SRP.panel2.N_hat
  Constant2 : Constant  Value=SRP.panel2.rho_s
  Constant3 : Constant  Value=SRP.panel2.rho_d
  A_i : Outport
  N_B_hat_i : Outport  Port=2
  rho_s_i : Outport  Port=3
  rho_d_i : Outport  Port=4
  wires:
  Constant3/1 -> rho_d_i/1
  Constant2/1 -> rho_s_i/1
  Constant1/1 -> N_B_hat_i/1
  Constant/1 -> A_i/1

== system SIM_SAD_DEMO/DKE/Earth radiation torque/Panel 3 ==
  Constant : Constant  Value=SRP.panel3.A
  Constant1 : Constant  Value=SRP.panel3.N_hat
  Constant2 : Constant  Value=SRP.panel3.rho_s
  Constant3 : Constant  Value=SRP.panel3.rho_d
  A_i : Outport
  N_B_hat_i : Outport  Port=2
  rho_s_i : Outport  Port=3
  rho_d_i : Outport  Port=4
  wires:
  Constant/1 -> A_i/1
  Constant1/1 -> N_B_hat_i/1
  Constant2/1 -> rho_s_i/1
  Constant3/1 -> rho_d_i/1

== system SIM_SAD_DEMO/DKE/Earth radiation torque/Panel 4 ==
  Constant : Constant  Value=SRP.panel4.A
  Constant1 : Constant  Value=SRP.panel4.N_hat
  Constant2 : Constant  Value=SRP.panel4.rho_s
  Constant3 : Constant  Value=SRP.panel4.rho_d
  A_i : Outport
  N_B_hat_i : Outport  Port=2
  rho_s_i : Outport  Port=3
  rho_d_i : Outport  Port=4
  wires:
  Constant3/1 -> rho_d_i/1
  Constant2/1 -> rho_s_i/1
  Constant1/1 -> N_B_hat_i/1
  Constant/1 -> A_i/1

== system SIM_SAD_DEMO/DKE/Earth-S//C Orbit/Conic Equation ==
  a : Inport
  e : Inport  Port=2
  theta_rad(t) : Inport  Port=3
  Constant : Constant  Value=2
  Constant1 : Constant
  Constant2 : Constant
  Cos : Trigonometry  Operator=cos
  Divide : Product  Inputs=*/
  Power : Math  Operator=pow
  Product : Product
  Product1 : Product
  Sum : Sum  Inputs=+-
  Sum1 : Sum
  r : Outport
  wires:
  a/1 -> Product/1
  e/1 -> Product1/1, Power/1
  Constant/1 -> Power/2
  Power/1 -> Sum/2
  Constant1/1 -> Sum/1
  Sum/1 -> Product/2
  Product/1 -> Divide/1
  Divide/1 -> r/1
  Constant2/1 -> Sum1/1
  theta_rad(t)/1 -> Cos/1
  Cos/1 -> Product1/2
  Product1/1 -> Sum1/2
  Sum1/1 -> Divide/2

== system SIM_SAD_DEMO/DKE/Earth-S//C Orbit/r (Inertial Frame) ==
  r : Inport
  theta_rad(t) : Inport  Port=2
  incl_rad : Inport  Port=3
  raan_rad : Inport  Port=4
  w_rad : Inport  Port=5
  Cos{,1..5} (6 alike) : Trigonometry  Operator=cos
  Product{,1,3,5} (4 alike) : Product
  Product2 : Product  Inputs=3
  Product4 : Product  Inputs=3
  Sin{,1..5} (6 alike) : Trigonometry
  Sum : Sum
  Sum1 : Sum  Inputs=+-
  Sum2 : Sum
  Vector Concatenate : Concatenate  NumInputs=3
  r_N : Outport
  wires:
  r/1 -> Product/1
  raan_rad/1 -> Cos/1, Cos4/1, Sin2/1, Sin/1
  w_rad/1 -> Sum/2
  Cos/1 -> Product1/2
  theta_rad(t)/1 -> Sum/1
  Sum/1 -> Sin4/1, Sin3/1, Cos3/1, Sin1/1, Cos1/1  "w+theta"
  Cos1/1 -> Product1/1
  Product1/1 -> Sum1/1
  Product2/1 -> Sum1/2
  Sin/1 -> Product2/1
  Sin1/1 -> Product2/2
  Cos2/1 -> Product2/3
  incl_rad/1 -> Cos5/1, Sin5/1, Cos2/1
  Sum1/1 -> Vector Concatenate/1
  Sum2/1 -> Vector Concatenate/2
  Sin2/1 -> Product3/1
  Cos3/1 -> Product3/2
  Product3/1 -> Sum2/1
  Product4/1 -> Sum2/2
  Cos4/1 -> Product4/1
  Sin3/1 -> Product4/2
  Cos5/1 -> Product4/3
  Sin4/1 -> Product5/1
  Sin5/1 -> Product5/2
  Product5/1 -> Vector Concatenate/3
  Vector Concatenate/1 -> Product/2
  Product/1 -> r_N/1

== system SIM_SAD_DEMO/DKE/Magnetic Torque/IGRF magnetic torque ==
  r_S/C_N : Inport
  Add : Sum  Inputs=+-
  Clock : Clock
  Constant : Constant  Value=JD0
  Constant2 : Constant  Value=Re
  Display{,1..3} (4 alike) : Display
  Gain : Gain  Gain=1000
  Gain1 : Gain  Gain=1000
  International Geomagnetic Reference Field : IGRF  time_in=off  month=January  day=1
      settings: AttributesFormatString=%<generation>
  MATLAB Function : MATLAB Function  TreatAsAtomicUnit=on
  MATLAB Function1 : MATLAB Function  TreatAsAtomicUnit=on
  MATLAB Function2 : MATLAB Function  TreatAsAtomicUnit=on
  MATLAB Function3 : LIBRARY_SAD/B_N (IGRF Model - Order N)/MATLAB Function3  SystemSampleTime=-1  VariantActivationTime=update diagram  EmptyChoice=off  PassThrough=off  PassThroughVariantControl=(default)  EmptyChoiceVariantControl=(default)  AllowFlexibleInterface=on  Latency=0  AutoFrameSizeCalculation=off
  Norm : Subsystem
  Scope : Scope
      settings: ActiveDisplayYMinimum=-1  ActiveDisplayYMaximum=1  DataLoggingVariableName=ScopeData23
  Scope1 : Scope
      settings: ActiveDisplayYMinimum=-1  ActiveDisplayYMaximum=1  DataLoggingVariableName=ScopeData24
  B_ECI : Outport
  wires:
  International Geomagnetic Reference Field/1 -> Scope1/1, MATLAB Function2/1(B_NED)
  MATLAB Function2/1(B_ECI) -> B_ECI/1
  Add/1 -> International Geomagnetic Reference Field/1, Display1/1
  Gain1/1 -> Add/1
  Clock/1 -> MATLAB Function/2(t), MATLAB Function2/4(t)
  MATLAB Function/1(r_ecef) -> MATLAB Function1/1(r_ecef)
  MATLAB Function1/1(lat) -> MATLAB Function2/2(lat_deg), Display2/1, International Geomagnetic Reference Field/2, Scope/1
  Gain/1 -> Add/2
  MATLAB Function1/2(lon) -> International Geomagnetic Reference Field/3, MATLAB Function2/3(lon_deg), Display3/1
  r_S/C_N/1 -> Norm/1(In1), MATLAB Function/1(r_eci)  "r_S/C_N"
  Constant/1 -> MATLAB Function3/1
  Norm/1(Out1) -> Gain1/1
  Constant2/1 -> Gain/1
  MATLAB Function3/1 -> MATLAB Function/3(alpha_G0), MATLAB Function2/5(alpha_G0), Display/1

== system SIM_SAD_DEMO/DKE/Solar Radiation Torque (SRP)/Body 1 ==
  Constant : Constant  Value=SRP.body1.A
  Constant1 : Constant  Value=SRP.body1.N_hat
  Constant2 : Constant  Value=SRP.body1.rho_s
  Constant3 : Constant  Value=SRP.body1.rho_d
  A_i : Outport
  N_B_hat_i : Outport  Port=2
  rho_s_i : Outport  Port=3
  rho_d_i : Outport  Port=4
  wires:
  Constant/1 -> A_i/1
  Constant1/1 -> N_B_hat_i/1
  Constant2/1 -> rho_s_i/1
  Constant3/1 -> rho_d_i/1

== system SIM_SAD_DEMO/DKE/Solar Radiation Torque (SRP)/Body 2 ==
  Constant : Constant  Value=SRP.body2.A
  Constant1 : Constant  Value=SRP.body2.N_hat
  Constant2 : Constant  Value=SRP.body2.rho_s
  Constant3 : Constant  Value=SRP.body2.rho_d
  A_i : Outport
  N_B_hat_i : Outport  Port=2
  rho_s_i : Outport  Port=3
  rho_d_i : Outport  Port=4
  wires:
  Constant3/1 -> rho_d_i/1
  Constant2/1 -> rho_s_i/1
  Constant1/1 -> N_B_hat_i/1
  Constant/1 -> A_i/1

== system SIM_SAD_DEMO/DKE/Solar Radiation Torque (SRP)/Body 3 ==
  Constant : Constant  Value=SRP.body3.A
  Constant1 : Constant  Value=SRP.body3.N_hat
  Constant2 : Constant  Value=SRP.body3.rho_s
  Constant3 : Constant  Value=SRP.body3.rho_d
  A_i : Outport
  N_B_hat_i : Outport  Port=2
  rho_s_i : Outport  Port=3
  rho_d_i : Outport  Port=4
  wires:
  Constant/1 -> A_i/1
  Constant1/1 -> N_B_hat_i/1
  Constant2/1 -> rho_s_i/1
  Constant3/1 -> rho_d_i/1

== system SIM_SAD_DEMO/DKE/Solar Radiation Torque (SRP)/Body 4 ==
  Constant : Constant  Value=SRP.body4.A
  Constant1 : Constant  Value=SRP.body4.N_hat
  Constant2 : Constant  Value=SRP.body4.rho_s
  Constant3 : Constant  Value=SRP.body4.rho_d
  A_i : Outport
  N_B_hat_i : Outport  Port=2
  rho_s_i : Outport  Port=3
  rho_d_i : Outport  Port=4
  wires:
  Constant3/1 -> rho_d_i/1
  Constant2/1 -> rho_s_i/1
  Constant1/1 -> N_B_hat_i/1
  Constant/1 -> A_i/1

== system SIM_SAD_DEMO/DKE/Solar Radiation Torque (SRP)/Body 5 ==
  Constant : Constant  Value=SRP.body5.A
  Constant1 : Constant  Value=SRP.body5.N_hat
  Constant2 : Constant  Value=SRP.body5.rho_s
  Constant3 : Constant  Value=SRP.body5.rho_d
  A_i : Outport
  N_B_hat_i : Outport  Port=2
  rho_s_i : Outport  Port=3
  rho_d_i : Outport  Port=4
  wires:
  Constant/1 -> A_i/1
  Constant1/1 -> N_B_hat_i/1
  Constant2/1 -> rho_s_i/1
  Constant3/1 -> rho_d_i/1

== system SIM_SAD_DEMO/DKE/Solar Radiation Torque (SRP)/Body 6 ==
  Constant : Constant  Value=SRP.body6.A
  Constant1 : Constant  Value=SRP.body6.N_hat
  Constant2 : Constant  Value=SRP.body6.rho_s
  Constant3 : Constant  Value=SRP.body6.rho_d
  A_i : Outport
  N_B_hat_i : Outport  Port=2
  rho_s_i : Outport  Port=3
  rho_d_i : Outport  Port=4
  wires:
  Constant3/1 -> rho_d_i/1
  Constant2/1 -> rho_s_i/1
  Constant1/1 -> N_B_hat_i/1
  Constant/1 -> A_i/1

== system SIM_SAD_DEMO/DKE/Solar Radiation Torque (SRP)/Panel 1 ==
  Constant : Constant  Value=SRP.panel1.A
  Constant1 : Constant  Value=SRP.panel1.N_hat
  Constant2 : Constant  Value=SRP.panel1.rho_s
  Constant3 : Constant  Value=SRP.panel1.rho_d
  A_i : Outport
  N_B_hat_i : Outport  Port=2
  rho_s_i : Outport  Port=3
  rho_d_i : Outport  Port=4
  wires:
  Constant/1 -> A_i/1
  Constant1/1 -> N_B_hat_i/1
  Constant2/1 -> rho_s_i/1
  Constant3/1 -> rho_d_i/1

== system SIM_SAD_DEMO/DKE/Solar Radiation Torque (SRP)/Panel 2 ==
  Constant : Constant  Value=SRP.panel2.A
  Constant1 : Constant  Value=SRP.panel2.N_hat
  Constant2 : Constant  Value=SRP.panel2.rho_s
  Constant3 : Constant  Value=SRP.panel2.rho_d
  A_i : Outport
  N_B_hat_i : Outport  Port=2
  rho_s_i : Outport  Port=3
  rho_d_i : Outport  Port=4
  wires:
  Constant3/1 -> rho_d_i/1
  Constant2/1 -> rho_s_i/1
  Constant1/1 -> N_B_hat_i/1
  Constant/1 -> A_i/1

== system SIM_SAD_DEMO/DKE/Solar Radiation Torque (SRP)/Panel 3 ==
  Constant : Constant  Value=SRP.panel3.A
  Constant1 : Constant  Value=SRP.panel3.N_hat
  Constant2 : Constant  Value=SRP.panel3.rho_s
  Constant3 : Constant  Value=SRP.panel3.rho_d
  A_i : Outport
  N_B_hat_i : Outport  Port=2
  rho_s_i : Outport  Port=3
  rho_d_i : Outport  Port=4
  wires:
  Constant/1 -> A_i/1
  Constant1/1 -> N_B_hat_i/1
  Constant2/1 -> rho_s_i/1
  Constant3/1 -> rho_d_i/1

== system SIM_SAD_DEMO/DKE/Solar Radiation Torque (SRP)/Panel 4 ==
  Constant : Constant  Value=SRP.panel4.A
  Constant1 : Constant  Value=SRP.panel4.N_hat
  Constant2 : Constant  Value=SRP.panel4.rho_s
  Constant3 : Constant  Value=SRP.panel4.rho_d
  A_i : Outport
  N_B_hat_i : Outport  Port=2
  rho_s_i : Outport  Port=3
  rho_d_i : Outport  Port=4
  wires:
  Constant3/1 -> rho_d_i/1
  Constant2/1 -> rho_s_i/1
  Constant1/1 -> N_B_hat_i/1
  Constant/1 -> A_i/1

== system SIM_SAD_DEMO/DKE/Magnetic Torque/IGRF magnetic torque/Norm ==
  note: square
  In1 : Inport
  Sqrt : Sqrt
  Square1 : Math  Operator=square
  Sum of Elements : Sum  Inputs=+
  Out1 : Outport
  wires:
  Square1/1 -> Sum of Elements/1
  Sqrt/1 -> Out1/1
  In1/1 -> Square1/1
  Sum of Elements/1 -> Sqrt/1

== matlab function SIM_SAD_DEMO/DKE/Magnetic Torque/IGRF magnetic torque/MATLAB Function ==
  data: r_eci input; r_ecef output; t input; alpha_G0 input
function r_ecef = eci2ecef(r_eci, t, alpha_G0)
% r_eci: [x, y, z] in meters (ECI frame)
% t: simulation time in seconds
% Default reference date: 1 Jan 2025 at 00:00 UTC

% Earth rotation rate (rad/s)
omega_earth = 7.2921159e-5;

% Compute Earth rotation angle
theta = alpha_G0 + omega_earth * t; % radians since reference epoch

% Rotation matrix about Z-axis
Rz = [cos(theta) sin(theta) 0;
     -sin(theta) cos(theta) 0;
      0          0          1];

% Convert ECI to ECEF
r_ecef = Rz * r_eci(:);
end
